simulink model "sim_Pendulum_TrolleyWithSwingingLoad"  (R2020a)
settings: Solver=VariableStepAuto  StartTime=0.0  StopTime=10  RelTol=1e-3
values from neighbouring files (symbols this model uses):
  a = 5    [Pendulum_TrolleyWithSwingingLoad.m]
  c = 200000    [Pendulum_TrolleyWithSwingingLoad.m]
  d_t = 1    [Pendulum_TrolleyWithSwingingLoad.m]
  F0 = 2000    [Pendulum_TrolleyWithSwingingLoad.m]
  g = 9.81    [Pendulum_TrolleyWithSwingingLoad.m]    (also in Pendulum_withFreeSupport.m = 9.8)
  J_l = 400    [Pendulum_TrolleyWithSwingingLoad.m]
  l = 4    [Pendulum_TrolleyWithSwingingLoad.m]    (also in Pendulum_withFreeSupport.m = 10)
  m_k = 100    [Pendulum_TrolleyWithSwingingLoad.m]
  m_l = 500    [Pendulum_TrolleyWithSwingingLoad.m]
settings Model: Creator=Samir  LastModifiedBy=Samir

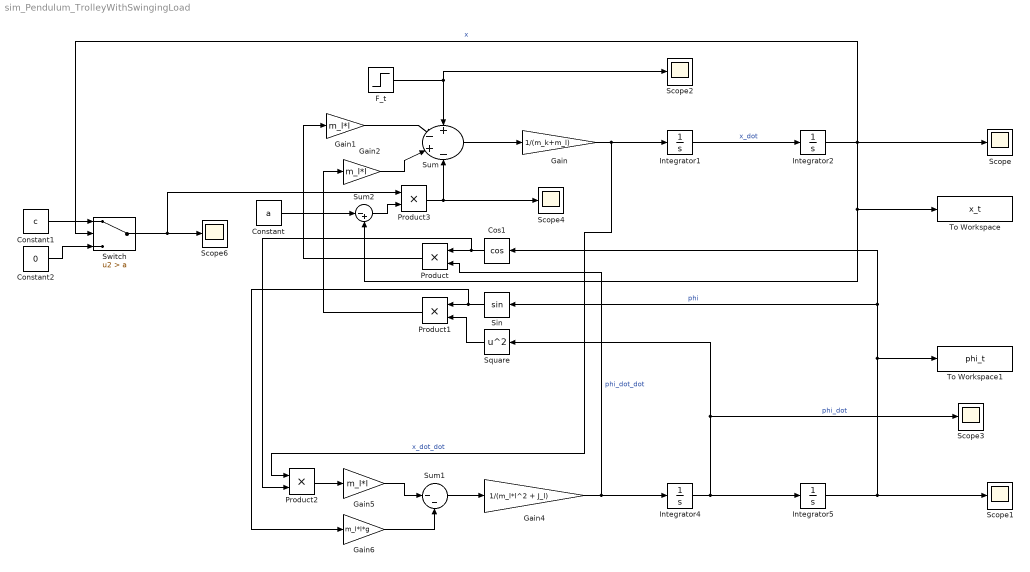
== system sim_Pendulum_TrolleyWithSwingingLoad ==
  Constant : Constant  Value=a
  Constant1 : Constant  Value=c
  Constant2 : Constant  Value=0
  Cos1 : Trigonometry  Operator=cos
  F_t : Step  Time=d_t  Before=F0  After=0  SampleTime=0
  Gain : Gain  Gain=1/(m_k+m_l)
  Gain1 : Gain  Gain=m_l*l
  Gain2 : Gain  Gain=m_l*l
  Gain4 : Gain  Gain=1/(m_l*l^2 + J_l)
  Gain5 : Gain  Gain=m_l*l
  Gain6 : Gain  Gain=m_l*l*g
  Integrator{1..2,4..5} (4 alike) : Integrator
  Product{,1..3} (4 alike) : Product
  Scope{,1..4,6} (6 alike) : Scope
  Sin : Trigonometry
  Square : Math  Operator=square  SaturateOnIntegerOverflow=on
  Sum : Sum  Inputs=+-+-
  Sum1 : Sum  Inputs=|--
  Sum2 : Sum  Inputs=|-+
  Switch : Switch  Criteria=u2 > Threshold  Threshold=a
  To Workspace : ToWorkspace  VariableName=x_t  SaveFormat=Timeseries  SampleTime=-1
  To Workspace1 : ToWorkspace  VariableName=phi_t  SaveFormat=Timeseries  SampleTime=-1
  wires:
  Gain/1 -> Product2/1, Integrator1/1  "x_dot_dot"
  Integrator1/1 -> Integrator2/1  "x_dot"
  Integrator4/1 -> Square/1, Scope3/1, Integrator5/1  "phi_dot"
  Gain4/1 -> Product/2, Integrator4/1  "phi_dot_dot"
  Integrator2/1 -> To Workspace/1, Sum2/2, Switch/2, Scope/1  "x"
  Sum/1 -> Gain/1
  F_t/1 -> Scope2/1, Sum/1
  Gain1/1 -> Sum/2
  Cos1/1 -> Product2/2, Product/1
  Product/1 -> Gain1/1
  Gain2/1 -> Sum/3
  Sin/1 -> Gain6/1, Product1/1
  Integrator5/1 -> To Workspace1/1, Sin/1, Cos1/1, Scope1/1  "phi"
  Square/1 -> Product1/2
  Product1/1 -> Gain2/1
  Constant/1 -> Sum2/1
  Sum2/1 -> Product3/2
  Product3/1 -> Sum/4, Scope4/1
  Sum1/1 -> Gain4/1
  Gain5/1 -> Sum1/1
  Product2/1 -> Gain5/1
  Gain6/1 -> Sum1/2
  Constant2/1 -> Switch/3
  Constant1/1 -> Switch/1
  Switch/1 -> Product3/1, Scope6/1
